simulink model "Three_Pools_Variable"  (Simulink 6.6)
settings: Solver=ode23tb  StartTime=0.0  StopTime=24  RelTol=1e-3
values from neighbouring files (symbols this model uses):
  sp = 1/max([f1, f2])/100    [GenPulses.m]
undefined symbols (not defined in the file or in its folder): C1, C2, C3, Library_RCelements, R, R1, R2, R3, R4, V3
libraries: simulink x3
settings Model: Creator=mladen  LastModifiedBy=mladen
settings OptimizationCC: BlockReduction=off  BooleanDataType=off
settings DebuggingCC: SignalResolutionControl=TryResolveAllWithWarning  SolverPrmCheckMsg=none  MultiTaskDSMMsg=warning  MultiTaskCondExecSysMsg=none  StrictBusMsg=None
settings HardwareCC: TargetUnknown=on
settings RTWCC: IncludeERTFirstTime=on
settings GRTTargetCC: ModelReferenceCompliant=off  MatFileLogging=off

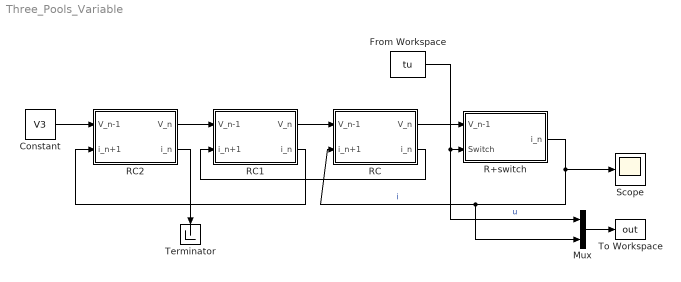
== system Three_Pools_Variable ==
  Constant : Constant  Value=V3
  From Workspace : FromWorkspace  VariableName=tu  SampleTime=sp  OutputAfterFinalValue=Holding final value
  Mux : Mux  Inputs=2
  R+switch : Subsystem  AncestorBlock=Library_RCelements/R+switch  mask(Switch plus Resistor){R1=R1}
      mask prompts: R1 "Resistance R"
      mask init:
      | x1 = [0.1 0.2 0.21:.02:0.43 0.44 0.6]+0.1;
      | y1= [0.8 0.8 0.85 0.75 0.85 0.75 0.85 0.75 0.85 0.75 0.85 0.75 0.85 0.75 0.80 0.80];
      | x2 = [0.2 0.7];
      | y2 = [0.2 0.2];
      | x3 = [0.7 0.7];
      | x4 = [0.7 0.7];
      | y3 = [0.8 0.6];
      | y4 = [0.45 0.2];
      | x5 = [0.7 0.77];
      | y5 = [0.6 0.4];
      mask Display:
      | plot(x1,y1, x2, y2);
      | plot(x3,y3);
      | plot(x4,y4);
      | plot(x5,y5);
  RC : Subsystem  AncestorBlock=Library_RCelements/RC  mask(Single RC){Rn=R2, Cn=C1, initVal=V3}
      mask prompts: Rn "Resistance"; Cn "Capacitance"; initVal "Initial Voltage accross the condensor"
      mask help: Single RC element
      mask init:
      | x1 = [0.1 0.2 0.21:.02:0.43 0.44 0.7]+0.1;
      | y1= [0.8 0.8 0.85 0.75 0.85 0.75 0.85 0.75 0.85 0.75 0.85 0.75 0.85 0.75 0.80 0.80];
      | x2 = [0.2 0.8];
      | y2 = [0.2 0.2];
      | x3 = [0.7 0.7];
      | x4 = [0.7 0.7];
      | y3 = [0.8 0.6];
      | y4 = [0.55 0.2];
      | x5 = [0.63 0.77];
      | y5 = [0.6 0.6];
      | x6 = [0.63 0.77];
      | y6 = [0.55 0.55];
      mask Display:
      | plot(x1,y1, x2, y2);
      | plot(x3,y3);
      | plot(x4,y4);
      | plot(x5,y5);
      | plot(x6,y6);
  RC1 : Subsystem  AncestorBlock=Library_RCelements/RC  mask(Single RC){Rn=R3, Cn=C2, initVal=V3}
      mask prompts: Rn "Resistance"; Cn "Capacitance"; initVal "Initial Voltage accross the condensor"
      mask help: Single RC element
      mask init: same as Three_Pools_Variable/RC
      mask Display:
      | plot(x1,y1, x2, y2);
      | plot(x3,y3);
      | plot(x4,y4);
      | plot(x5,y5);
      | plot(x6,y6);
  RC2 : Subsystem  AncestorBlock=Library_RCelements/RC  mask(Single RC){Rn=R4, Cn=C3, initVal=V3}
      mask prompts: Rn "Resistance"; Cn "Capacitance"; initVal "Initial Voltage accross the condensor"
      mask help: Single RC element
      mask init: same as Three_Pools_Variable/RC
      mask Display:
      | plot(x1,y1, x2, y2);
      | plot(x3,y3);
      | plot(x4,y4);
      | plot(x5,y5);
      | plot(x6,y6);
  Scope : Scope
  Terminator : Terminator
      settings: Orientation=down
  To Workspace : ToWorkspace  VariableName=out  SampleTime=sp  SaveFormat=Structure With Time
  wires:
  RC/1(V_n) -> R+switch/1(V_n-1)
  R+switch/1(i_n) -> Mux/2, RC/2(i_n+1), Scope/1  "i"
  RC1/1(V_n) -> RC/1(V_n-1)
  Constant/1 -> RC2/1(V_n-1)
  RC/2(i_n) -> RC1/2(i_n+1)
  RC1/2(i_n) -> RC2/2(i_n+1)
  Mux/1 -> To Workspace/1
  From Workspace/1 -> R+switch/2(Switch), Mux/1  "u"
  RC2/1(V_n) -> RC1/1(V_n-1)
  RC2/2(i_n) -> Terminator/1

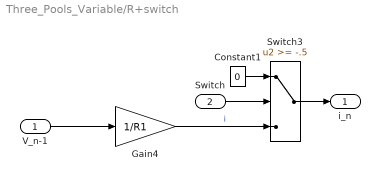
== system Three_Pools_Variable/R+switch ==
  V_n-1 : Inport
  Switch : Inport  Port=2
  Constant1 : Constant  Value=0
  Gain4 : Gain  Gain=1/R1  SaturateOnIntegerOverflow=on
  Switch3 : Switch  Threshold=-.5  SaturateOnIntegerOverflow=on  InputSameDT=on
  i_n : Outport
  wires:
  Constant1/1 -> Switch3/1
  Switch/1 -> Switch3/2
  Gain4/1 -> Switch3/3  "i"
  Switch3/1 -> i_n/1
  V_n-1/1 -> Gain4/1

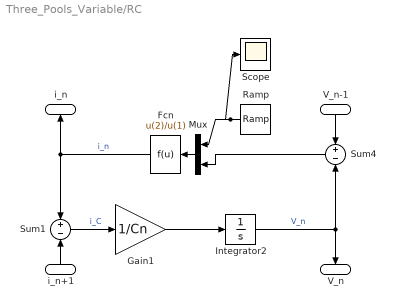
== system Three_Pools_Variable/RC ==
  V_n-1 : Inport  Orientation=down
  i_n+1 : Inport  Orientation=up  Port=2
  Fcn : Fcn  Orientation=left  Expr=u(2)/u(1)
  Gain1 : Gain  Gain=1/Cn  SaturateOnIntegerOverflow=on
  Integrator2 : Integrator  InitialCondition=initVal
  Mux : Mux  Orientation=left  Inputs=2
  Ramp : simulink/Sources/Ramp  Orientation=left  SystemSampleTime=-1  slope=1  start=1  X0=Rn
  Scope : Scope
  Sum1 : Sum  Inputs=+-  SaturateOnIntegerOverflow=on  InputSameDT=on
  Sum4 : Sum  Orientation=left  Inputs=+-  SaturateOnIntegerOverflow=on  InputSameDT=on
  V_n : Outport  Orientation=down
  i_n : Outport  Orientation=up  Port=2
  wires:
  V_n-1/1 -> Sum4/1
  Integrator2/1 -> Sum4/2, V_n/1  "V_n"
  Fcn/1 -> Sum1/1, i_n/1  "i_n"
  i_n+1/1 -> Sum1/2
  Sum1/1 -> Gain1/1  "i_C"
  Gain1/1 -> Integrator2/1
  Mux/1 -> Fcn/1
  Ramp/1 -> Mux/1, Scope/1
  Sum4/1 -> Mux/2

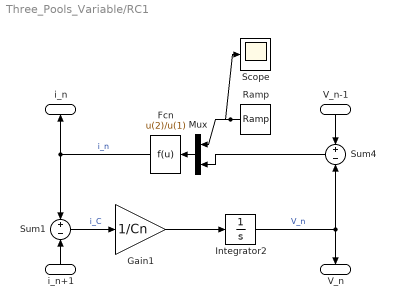
== system Three_Pools_Variable/RC1 ==
  V_n-1 : Inport  Orientation=down
  i_n+1 : Inport  Orientation=up  Port=2
  Fcn : Fcn  Orientation=left  Expr=u(2)/u(1)
  Gain1 : Gain  Gain=1/Cn  SaturateOnIntegerOverflow=on
  Integrator2 : Integrator  InitialCondition=initVal
  Mux : Mux  Orientation=left  Inputs=2
  Ramp : simulink/Sources/Ramp  Orientation=left  SystemSampleTime=-1  slope=1  start=1  X0=Rn
  Scope : Scope
  Sum1 : Sum  Inputs=+-  SaturateOnIntegerOverflow=on  InputSameDT=on
  Sum4 : Sum  Orientation=left  Inputs=+-  SaturateOnIntegerOverflow=on  InputSameDT=on
  V_n : Outport  Orientation=down
  i_n : Outport  Orientation=up  Port=2
  wires:
  V_n-1/1 -> Sum4/1
  Integrator2/1 -> Sum4/2, V_n/1  "V_n"
  Fcn/1 -> Sum1/1, i_n/1  "i_n"
  i_n+1/1 -> Sum1/2
  Sum1/1 -> Gain1/1  "i_C"
  Gain1/1 -> Integrator2/1
  Mux/1 -> Fcn/1
  Ramp/1 -> Mux/1, Scope/1
  Sum4/1 -> Mux/2

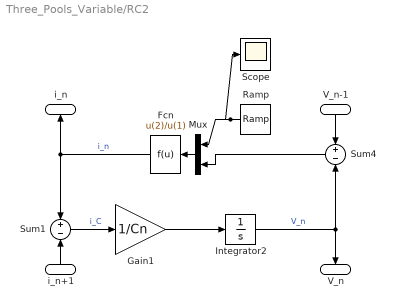
== system Three_Pools_Variable/RC2 ==
  V_n-1 : Inport  Orientation=down
  i_n+1 : Inport  Orientation=up  Port=2
  Fcn : Fcn  Orientation=left  Expr=u(2)/u(1)
  Gain1 : Gain  Gain=1/Cn  SaturateOnIntegerOverflow=on
  Integrator2 : Integrator  InitialCondition=initVal
  Mux : Mux  Orientation=left  Inputs=2
  Ramp : simulink/Sources/Ramp  Orientation=left  SystemSampleTime=-1  slope=1  start=1  X0=Rn
  Scope : Scope
  Sum1 : Sum  Inputs=+-  SaturateOnIntegerOverflow=on  InputSameDT=on
  Sum4 : Sum  Orientation=left  Inputs=+-  SaturateOnIntegerOverflow=on  InputSameDT=on
  V_n : Outport  Orientation=down
  i_n : Outport  Orientation=up  Port=2
  wires:
  V_n-1/1 -> Sum4/1
  Integrator2/1 -> Sum4/2, V_n/1  "V_n"
  Fcn/1 -> Sum1/1, i_n/1  "i_n"
  i_n+1/1 -> Sum1/2
  Sum1/1 -> Gain1/1  "i_C"
  Gain1/1 -> Integrator2/1
  Mux/1 -> Fcn/1
  Ramp/1 -> Mux/1, Scope/1
  Sum4/1 -> Mux/2
